simulink library "myLibrary"  (R2023a)
settings: Solver=VariableStepAuto  StartTime=0.0  StopTime=10.0  RelTol=1e-3
undefined symbols (not defined in the file): Cac_n1, ctrl1, Da, Discrete, dtha, ee_sli_rtmsupport, FA, gcbh, Ha, Ini, init_line, init_load, init_SG, init_TH, init_trafo, init_VSC, initMachineBlocks, Ka, Lf, Llkd_pu, Llkq1_pu, NET, P, plots_step, q0, Rac_n1, Radd, Rkd_pu, Rkq1_pu, Rload_add, sim_config, spsSteamTurbineModel, T_global, T_load, T_NET, T_SG, T_TH, T_trafo, T_VSC, Ts, tstep, V1
libraries: spsSeriesRLCBranchLib x57, spsParallelRLCBranchLib x39, eeGeneralControl x38, spsCurrentMeasurementLib x20, spsFirstOrderFilterLib x16, spsVoltageMeasurementLib x14, spsControlledVoltageSourceLib x12, $bdroot x9, dspsigops x6, spsThreePhaseVIMeasurementLib x5, spsPLL3phLib x4, spsThreePhaseBreakerLib x3
(part 3 of 7)

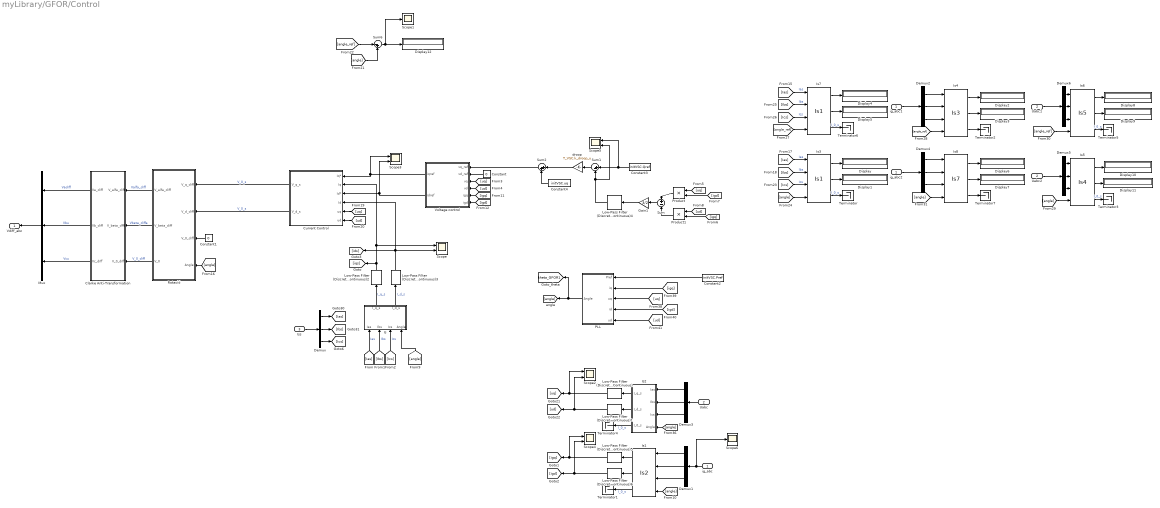
== system myLibrary/GFOR/Control ==
  ig_abc : Inport
  Uabc : Inport  Port=2
  Iss : Inport  Port=3
  Clarke Anti-Transformation : Subsystem
  Constant : Constant  Value=0
  Constant1 : Constant  Value=0
  Constant2 : Constant  Value=initVSC.Pref
  Constant3 : Constant  Value=initVSC.Qref
  Constant4 : Constant  Value=initVSC.uq
  Current Control : Subsystem
  Demux{,1..6} (7 alike) : Demux  Outputs=3
  Display{,1..12} (13 alike) : Display
  Gain1 : Gain  Gain=3/2
  Is : Subsystem
  Is1 : $bdroot/GFOR/Control/Is2  SystemSampleTime=-1  VariantActivationTime=update diagram  Latency=0  AutoFrameSizeCalculation=off
  Is2 : Subsystem
  Is3 : $bdroot/GFOL/Control/Is1  SystemSampleTime=-1  VariantActivationTime=update diagram  Latency=0  AutoFrameSizeCalculation=off
  Is4 : $bdroot/GFOL/Control/Is3  SystemSampleTime=-1  VariantActivationTime=update diagram  Latency=0  AutoFrameSizeCalculation=off
  Is5 : $bdroot/GFOL/Control/Is4  SystemSampleTime=-1  VariantActivationTime=update diagram  Latency=0  AutoFrameSizeCalculation=off
  Is6 : $bdroot/GFOL/Control/Is5  SystemSampleTime=-1  VariantActivationTime=update diagram  Latency=0  AutoFrameSizeCalculation=off
  Is7 : $bdroot/GFOL/Control/Is1  SystemSampleTime=-1  VariantActivationTime=update diagram  Latency=0  AutoFrameSizeCalculation=off
  Is8 : $bdroot/GFOL/Control/Is7  SystemSampleTime=-1  VariantActivationTime=update diagram  Latency=0  AutoFrameSizeCalculation=off
  Low-Pass Filter (Discrete or Continuous) : eeGeneralControl/Low-Pass Filter (Discrete or Continuous)  K=1  T=init_VSC.delay  B=inf  A=-inf  init_option=Specify as parameter  x0=initVSC.uq  Ts=0
  Low-Pass Filter (Discrete or Continuous)1 : eeGeneralControl/Low-Pass Filter (Discrete or Continuous)  K=1  T=init_VSC.delay  B=inf  A=-inf  init_option=Specify as parameter  x0=initVSC.ud  Ts=0
  Low-Pass Filter (Discrete or Continuous)2 : eeGeneralControl/Low-Pass Filter (Discrete or Continuous)  K=1  T=init_VSC.delay  B=inf  A=-inf  init_option=Specify as parameter  x0=initVSC.idiffq  Ts=0
  Low-Pass Filter (Discrete or Continuous)3 : eeGeneralControl/Low-Pass Filter (Discrete or Continuous)  K=1  T=init_VSC.delay  B=inf  A=-inf  init_option=Specify as parameter  x0=initVSC.idiffd  Ts=0
  Low-Pass Filter (Discrete or Continuous)4 : eeGeneralControl/Low-Pass Filter (Discrete or Continuous)  K=1  T=T_VSC.tau_droop_u  B=inf  A=-inf  init_option=Specify as parameter  x0=initVSC.Qref  Ts=0
  Low-Pass Filter (Discrete or Continuous)5 : eeGeneralControl/Low-Pass Filter (Discrete or Continuous)  K=1  T=init_VSC.delay  B=inf  A=-inf  init_option=Specify as parameter  x0=initVSC.igq  Ts=0
  Low-Pass Filter (Discrete or Continuous)6 : eeGeneralControl/Low-Pass Filter (Discrete or Continuous)  K=1  T=init_VSC.delay  B=inf  A=-inf  init_option=Specify as parameter  x0=initVSC.igd  Ts=0
  Mux : Mux  Inputs=3
  PLL : Subsystem
  Product : Product
  Product1 : Product
  Rotació : Subsystem
  Scope{,2..5} (5 alike) : Scope  NumInputPorts=2
  Scope1 : Scope
  Scope6 : Scope
  Sum : Sum  Inputs=+-
  Sum1 : Sum  Inputs=|+-
  Sum2 : Sum  Inputs=|++
  Sum6 : Sum  Inputs=|-+
  Terminator{,1..7} (8 alike) : Terminator
  Uabc1 : InportShadow  Port=2
  Uabc2 : InportShadow  Port=2
  Voltage control : Subsystem
  droop : Gain  Gain=T_VSC.k_droop_u
  ig_abc1 : InportShadow
  ig_abc2 : InportShadow
  Vdiff_abc : Outport
  tag scope: theta_GFOR1=global
  wires:
  Constant1/1 -> Rotació/3(V_0_diff)
  Low-Pass Filter (Discrete or Continuous)2/1 -> [iqs], Scope/1, Current Control/2(Iq)
  Low-Pass Filter (Discrete or Continuous)3/1 -> [ids], Current Control/4(Id), Scope/2
  Mux/1 -> Vdiff_abc/1
  Clarke Anti-Transformation/2(Vb_diff) -> Mux/2  "Vbu"
  Clarke Anti-Transformation/3(Vc_diff) -> Mux/3  "Vcu"
  Rotació/3(V_0) -> Clarke Anti-Transformation/3(V_0_diff)  "V_0_diff"
  Clarke Anti-Transformation/1(Va_diff) -> Mux/1  "Vadiff"
  Rotació/2(V_beta_diff) -> Clarke Anti-Transformation/2(V_beta_dfff)  "Vbeta_diffa"
  Rotació/1(V_alfa_diff) -> Clarke Anti-Transformation/1(V_alfa_diff)  "Valfa_diff"
  [angle_ref] -> Sum6/1
  Sum6/1 -> Display12/1, Scope1/1
  [angle] -> Sum6/2
  [ud] -> Current Control/6(ud)
  [uq] -> Current Control/5(uq)
  Current Control/2(V_d_s) -> Rotació/2(V_d_diff)  "V_0_s"
  Current Control/1(V_q_s) -> Rotació/1(V_q_diff)  "V_0_s"
  [angle] -> Rotació/4(Angle)
  [angle] -> Is/4(Angle)
  Iss/1 -> Demux/1
  Demux/3 -> [Ics]
  Demux/2 -> [Ibs]
  Demux/1 -> [Ias]
  [Ibs] -> Is/2(Ibs)  "Ibs"
  [Ics] -> Is/3(Ics)  "Ics"
  [Ias] -> Is/1(Ias)  "Ias"
  Is/1(I_q_s) -> Low-Pass Filter (Discrete or Continuous)2/1  "I_q_s"
  Is/2(I_d_s) -> Low-Pass Filter (Discrete or Continuous)3/1  "I_d_s"
  Constant/1 -> Voltage control/2(vd_ref)
  [igq] -> PLL/2(iq)
  Demux3/3 -> Is2/3(Ics)
  Demux3/2 -> Is2/2(Ibs)
  [angle] -> Is2/4(Angle)
  PLL/1(Angle) -> [theta_GFOR1], [angle]
  [uq] -> Voltage control/3(vq)
  [igd] -> PLL/4(id)
  Demux3/1 -> Is2/1(Ias)
  Low-Pass Filter (Discrete or Continuous)/1 -> Scope2/1, [uq]
  [uq] -> PLL/3(uq)
  Sum2/1 -> Voltage control/1(vq_ref)
  Constant2/1 -> PLL/1(Pref)
  [ud] -> Voltage control/4(vd)
  Low-Pass Filter (Discrete or Continuous)1/1 -> [ud], Scope2/2
  Is2/3(I_0_s) -> Terminator4/1  "I_0_s"
  Is2/2(I_d_s) -> Low-Pass Filter (Discrete or Continuous)1/1
  Uabc/1 -> Demux3/1
  Is2/1(I_q_s) -> Low-Pass Filter (Discrete or Continuous)/1
  [ud] -> PLL/5(ud)
  Voltage control/1(iqref) -> Current Control/1(Iq*), Scope3/1
  Voltage control/2(idref) -> Scope3/2, Current Control/3(Id*)
  [igd] -> Product/2
  Constant3/1 -> Sum1/1, Scope5/1
  Gain1/1 -> Low-Pass Filter (Discrete or Continuous)4/1
  Product1/1 -> Sum/2
  Product/1 -> Sum/1
  Sum/1 -> Gain1/1
  [igq] -> Product1/2
  Constant4/1 -> Sum2/2
  Sum1/1 -> droop/1
  [uq] -> Product/1
  [ud] -> Product1/1
  droop/1 -> Sum2/1
  Low-Pass Filter (Discrete or Continuous)4/1 -> Sum1/2, Scope5/2
  Low-Pass Filter (Discrete or Continuous)5/1 -> Scope4/1, [igq]
  Demux1/1 -> Is1/1
  Demux1/3 -> Is1/3
  ig_abc/1 -> Demux1/1, Scope6/1
  Is1/3 -> Terminator1/1  "I_0_s"
  Demux1/2 -> Is1/2
  Is1/2 -> Low-Pass Filter (Discrete or Continuous)6/1
  [angle] -> Is1/4
  Low-Pass Filter (Discrete or Continuous)6/1 -> [igd], Scope4/2
  Is1/1 -> Low-Pass Filter (Discrete or Continuous)5/1
  [igq] -> Voltage control/5(igq)
  [igd] -> Voltage control/6(igd)
  [angle] -> Is8/4
  Is4/2 -> Display3/1
  Is8/1 -> Display6/1
  Demux5/1 -> Is5/1
  [Ics] -> Is3/3  "Ics"
  Is8/3 -> Terminator7/1
  Uabc2/1 -> Demux5/1
  Demux2/3 -> Is4/3
  Demux2/1 -> Is4/1
  Is5/2 -> Display11/1
  Demux6/1 -> Is6/1
  Is5/3 -> Terminator3/1  "I_0_s"
  Demux6/3 -> Is6/3
  Is4/1 -> Display2/1
  ig_abc1/1 -> Demux2/1
  Demux4/3 -> Is8/3
  [Ias] -> Is7/1  "Ias"
  [Ibs] -> Is7/2  "Ibs"
  Demux5/2 -> Is5/2
  ig_abc2/1 -> Demux4/1
  Demux5/3 -> Is5/3
  Is7/3 -> Terminator6/1  "I_0_s"
  [angle_ref] -> Is4/4
  Is3/1 -> Display/1
  [Ics] -> Is7/3  "Ics"
  [angle_ref] -> Is7/4
  Is8/2 -> Display7/1
  Is7/2 -> Display5/1
  Is6/1 -> Display8/1
  Demux2/2 -> Is4/2
  [angle_ref] -> Is6/4
  [angle] -> Is3/4
  Is6/3 -> Terminator5/1  "I_0_s"
  Is4/3 -> Terminator2/1
  Is5/1 -> Display10/1
  Is7/1 -> Display4/1
  Demux4/1 -> Is8/1
  [Ias] -> Is3/1  "Ias"
  [Ibs] -> Is3/2  "Ibs"
  Is3/2 -> Display1/1
  Uabc1/1 -> Demux6/1
  Is6/2 -> Display9/1
  [angle] -> Is5/4
  Demux6/2 -> Is6/2
  Demux4/2 -> Is8/2
  Is3/3 -> Terminator/1  "I_0_s"

== system myLibrary/GFOR/Electrical ==
  note: DIFF CIRCUIT:
  Vdiff : Inport
  Controlled Voltage Source1 : spsControlledVoltageSourceLib/Controlled Voltage Source  Initialize=on  Source_Type=AC  Amplitude=initVSC.Udiff_mag  Phase=initVSC.angle_vdiff*180/pi  Frequency=T_VSC.fb  Measurements=None
  Controlled Voltage Source2 : spsControlledVoltageSourceLib/Controlled Voltage Source  Initialize=on  Source_Type=AC  Amplitude=initVSC.Udiff_mag  Phase=(initVSC.angle_vdiff -2*pi/3)*180/pi  Frequency=T_VSC.fb  Measurements=None
  Controlled Voltage Source3 : spsControlledVoltageSourceLib/Controlled Voltage Source  Initialize=on  Source_Type=AC  Amplitude=initVSC.Udiff_mag  Phase=(initVSC.angle_vdiff +2*pi/3)*180/pi  Frequency=T_VSC.fb  Measurements=None
  Demux : Demux  Outputs=3
  Mesura Ias10 : spsCurrentMeasurementLib/Current Measurement  PhasorSimulation=off  OutputType=Complex  PSBequivalent=0
  Mesura Ias7 : spsCurrentMeasurementLib/Current Measurement  PhasorSimulation=off  OutputType=Complex  PSBequivalent=0
  Mesura Ias9 : spsCurrentMeasurementLib/Current Measurement  PhasorSimulation=off  OutputType=Complex  PSBequivalent=0
  Mux : Mux  Inputs=3
  Scope : Scope
  Scope10 : Scope  NumInputPorts=3
  Zsa : spsSeriesRLCBranchLib/Series RLC Branch  LConnTagsString=__new0  RConnTagsString=__new0  BranchType=RL  Resistance=initVSC.Rc  Inductance=initVSC.Lc  SetiL0=off  InitialCurrent=initVSC.Isa  Capacitance=1e-6  Setx0=off  InitialVoltage=0  Measurements=None
  Zsa1 : spsSeriesRLCBranchLib/Series RLC Branch  LConnTagsString=__new0  RConnTagsString=__new0  BranchType=RL  Resistance=initVSC.Rc  Inductance=initVSC.Lc  SetiL0=on  InitialCurrent=initVSC.Isb  Capacitance=1e-6  Setx0=off  InitialVoltage=0  Measurements=None
  Zsa2 : spsSeriesRLCBranchLib/Series RLC Branch  LConnTagsString=__new0  RConnTagsString=__new0  BranchType=RL  Resistance=initVSC.Rc  Inductance=initVSC.Lc  SetiL0=on  InitialCurrent=initVSC.Isc  Capacitance=1e-6  Setx0=off  InitialVoltage=0  Measurements=None
  VA : PMIOPort  Side=Left
  VB : PMIOPort  Port=2  Side=Left
  VC : PMIOPort  Port=3  Side=Left
  Is : Outport
  wires:
  Mesura Ias10/1 -> [Ics]
  Mesura Ias7/1 -> [Ias]
  Mesura Ias9/1 -> [Ibs]
  Vdiff/1 -> Demux/1
  Demux/1 -> [Vdiffa]
  Demux/3 -> [Vdiffc]
  Demux/2 -> [Vdiffb]
  Mux/1 -> Scope/1, Is/1
  [Ics] -> Mux/3  "Ics"
  [Ibs] -> Mux/2  "Ibs"
  [Ias] -> Mux/1  "Ias"
  [Vdiffa] -> Controlled Voltage Source1/1, Scope10/1
  [Vdiffb] -> Scope10/2, Controlled Voltage Source2/1
  [Vdiffc] -> Controlled Voltage Source3/1, Scope10/3
  connections:
  Zsa1/LConn1 -- Controlled Voltage Source2/RConn1
  Mesura Ias7/RConn1 -- VA/RConn1
  Mesura Ias9/RConn1 -- VB/RConn1
  Mesura Ias10/RConn1 -- VC/RConn1
  Zsa/RConn1 -- Mesura Ias7/LConn1
  Zsa1/RConn1 -- Mesura Ias9/LConn1
  Zsa2/RConn1 -- Mesura Ias10/LConn1
  Controlled Voltage Source1/RConn1 -- Zsa/LConn1
  Zsa2/LConn1 -- Controlled Voltage Source3/RConn1
  Controlled Voltage Source3/LConn1 -- Controlled Voltage Source1/LConn1 -- Controlled Voltage Source2/LConn1

== system myLibrary/SG/Exciter ==
  V_REF : Inport
  Vq : Inport  Port=2
  Vd : Inport  Port=3
  Vsi1 : Inport  Port=4
  Vsi2 : Inport  Port=5
  Ifd_pu : Inport  Port=6
  Efd0_pu : Inport  Port=7
  Constant : Constant  Value=hasPSS
  Constant1 : Constant  Value=selectExciter
  Constant4 : Constant
  Constant5 : Constant  Value=initSG.Pm
  Exciter AC4A : Subsystem
  Exciter ST1 : Subsystem  Commented=on
  Exciter ST4B : Subsystem  Commented=on  AncestorBlock=eeSmST4C/SM ST4C  LoadFcn=ee_sli_rtmsupport( 'loadfcn', gcbh );  mask(SM ST4C){E_FD0=1, V_T0=1, I_T0=1, Ts=-1, T_R=T_SG.exc.TR, K_PR=T_SG.exc.KPR, K_IR=T_SG.exc.KIR, T_A=T_SG.exc.TA, K_PM=T_SG.exc.KPM, K_IM=T_SG.exc.KIM, K_G=T_SG.exc.KG, T_G=0, K_C=T_SG.exc.KC, K_P=T_SG.exc.KP, K_I=T_SG.exc.KI, X_L=T_SG.exc.XL, theta_P=0}
      mask prompts: E_FD0 "physmod:ee:library:comments:control:eeSmST4C:InitialFieldVoltageEfd0pu_MP"; V_T0 "physmod:ee:library:comments:control:eeSmST4C:InitialTerminalVoltageVt0pu_MP"; I_T0 "physmod:ee:library:comments:control:eeSmST4C:InitialTerminalCurrentIt0pu_MP"; Ts "physmod:ee:library:comments:control:eeSmST4C:SampleTime1ForInherited_MP"; T_R "physmod:ee:library:comments:control:eeSmST4C:RegulatorInputFilterTimeConstantT_Rs_MP"; K_PR "physmod:ee:library:comments:control:eeSmST4C:VoltageRegulatorProportionalGainK_PRpu_MP"; K_IR "physmod:ee:library:comments:control:eeSmST4C:VoltageRegulatorIntegralGainK_IRpus_MP"; T_A "physmod:ee:library:comments:control:eeSmST4C:ThyristorBridgeFiringControlEquivalentTimeConstantT_As_MP"; K_PM "physmod:ee:library:comments:control:eeSmST4C:ForwardProportionalGainOfInnerLoopFieldRegulatorK_PMpu_MP"; K_IM "physmod:ee:library:comments:control:eeSmST4C:ForwardIntegralGainOfInnerLoopFieldRegulatorK_IMpus_MP"; K_G "physmod:ee:library:comments:control:eeSmST4C:FeedbackGainOfFieldCurrentRegulatorK_Gpu_MP"; T_G "physmod:ee:library:comments:control:eeSmST4C:FeedbackTimeConstantOfFieldCurrentRegulatorT_Gs_MP"; K_C "physmod:ee:library:comments:control:eeSmST4C:RectifierLoadingFactorProportionalToCommutatingReactanceK_Cp_MP"; K_P "physmod:ee:library:comments:control:eeSmST4C:PotentialCircuitvoltageGainCoefficientK_Ppu_MP"; K_I "physmod:ee:library:comments:control:eeSmST4C:CompoundCircuitcurrentGainCoefficientK_Ipu_MP"; X_L "physmod:ee:library:comments:control:eeSmST4C:ReactanceAssociatedWithPotentialSourceX_Lpu_MP"; theta_P "physmod:ee:library:comments:control:eeSmST4C:PotentialCircuitPhaseAngledegrees_MP"
      mask help: physmod:ee:library:comments:control:eeSmST4C:SMST4C_MD
      mask init:
      | %[timeDomain,isVsSummationPoint1,isVsSummationPoint2,...
      | %    isOelSummationPoint,isOelTakeOver1,isOelTakeOver2,...
      | %    isUelSummationPoint,isUelTakeOver1,isUelTakeOver2,...
      | %    isSclSummationPoint,isSclTakeOver1,isSclTakeOver2,isSw1LocationA]...
      | %    = ee.mask.initializeST4C(Ts,oelInputLocation,...
      | %    uelInputLocation,sclInputLocation,vsInputLocation,SW1);
      | 
      | %This will move to Initialization Function
      | %[V_G0,initialOffset] = ee.control.sm.initializeST4C(E_FD0,V_T0,I_T0,K_G,theta_P,K_P,X_L,K_I,K_C,V_Bmax,SW1);
      settings: LibrarySourceBlock=eeSmST4C/SM ST4C  CopyFcn=ee_sli_rtmsupport( 'copyfcn', gcbh );  DeleteFcn=ee_sli_rtmsupport( 'deletefcn', gcbh );  ModelCloseFcn=ee_sli_rtmsupport( 'modelclosefcn', gcbh );  PostSaveFcn=ee_sli_rtmsupport( 'postsavefcn', gcbh );  PreCopyFcn=ee_sli_rtmsupport( 'precopyfcn', gcbh );  OpenFcn=ee_sli_rtmsupport( 'openfcn', gcbh );  CloseFcn=ee_sli_rtmsupport( 'closefcn', gcbh );  PreDeleteFcn=ee_sli_rtmsupport( 'predeletefcn', gcbh );
      mask Help: web(nesl_help(gcbh))
      mask TypeOptions Ts:
      | Voltage Transducer/Ts | PI_R/Integrator
      | (Discrete or Continuous)/Ts | PI_M/Integrator
      | (Discrete or Continuous)/Ts | VRminmax/Ts | K_G//(1+sT_G)/Ts
      mask DialogControl TabGeneral Prompt: physmod:ee:library:comments:control:eeSmST4C:tab_General
      mask DialogControl E_FD0 Prompt: Initial field voltage, Efd0 (pu)
      mask DialogControl V_T0 Prompt: Initial terminal voltage, Vt0 (pu)
      mask DialogControl I_T0 Prompt: Initial terminal current, It0 (pu)
      mask DialogControl Ts Prompt: Sample time (-1 for inherited)
      mask DialogControl TabPrecontrol Prompt: physmod:ee:library:comments:control:eeSmST4C:tab_PreControl
      mask DialogControl T_R Prompt: Regulator input filter time constant, T_R (s)
      mask DialogControl TabControl Prompt: physmod:ee:library:comments:control:eeSmST4C:tab_Control
      mask DialogControl K_PR Prompt: Voltage regulator proportional gain, K_PR (pu)
      mask DialogControl K_IR Prompt: Voltage regulator integral gain, K_IR (pu/s)
      mask DialogControl T_A Prompt: Thyristor bridge firing control equivalent time constant, T_A (s)
      mask DialogControl K_PM Prompt: Forward proportional gain of inner loop field regulator, K_PM (pu)
      mask DialogControl K_IM Prompt: Forward integral gain of inner loop field regulator, K_IM (pu/s)
      mask DialogControl K_G Prompt: Feedback gain of field current regulator, K_G (pu)
      mask DialogControl T_G Prompt: Feedback time constant of field current regulator, T_G (s)
      mask DialogControl TabExciter Prompt: physmod:ee:library:comments:control:eeSmST4C:tab_Exciter
      mask DialogControl K_C Prompt: Rectifier loading factor proportional to commutating reactance, K_C (pu)
      mask DialogControl K_P Prompt: Potential circuit (voltage) gain coefficient, K_P (pu)
      mask DialogControl K_I Prompt: Compound circuit (current) gain coefficient, K_I (pu)
      mask DialogControl X_L Prompt: Reactance associated with potential source, X_L (pu)
      mask DialogControl theta_P Prompt: Potential circuit phase angle (degrees)
      mask Display: %ee.mask.drawSTxC(gcb);
  Gain : Gain  Gain=T_SG.Lmd_pu
  Multiport Switch : MultiPortSwitch  Inputs=4  SaturateOnIntegerOverflow=off  InputSameDT=off
  PSS 2A : Subsystem  Commented=on  mask{ks1=T_SG.PSS.Ks1, ks2=T_SG.PSS.Ks2, ks3=T_SG.PSS.Ks3, T6=T_SG.PSS.T6, T7=T_SG.PSS.T7, Tw1=T_SG.PSS.Tw1, Tw2=T_SG.PSS.Tw2, Tw3=T_SG.PSS.Tw3, Tw4=T_SG.PSS.Tw4, T8=T_SG.PSS.T8, T9=T_SG.PSS.T9, M=T_SG.PSS.M, N=T_SG.PSS.N, T1=T_SG.PSS.T1, T2=T_SG.PSS.T2, T3=T_SG.PSS.T3, T4=T_SG.PSS.T4, hasPSS=hasPSS}
      mask prompts: ks1 "PSS gain, K_S1 (pu)"; ks2 "PSS gain, K_S2 (pu)"; ks3 "PSS gain, K_S3 (pu)"; T6 "PSS transducer time constant, T_6 (s)"; T7 "PSS transducer time constant, T_7 (s)"; Tw1 "PSS washout time constant, T_w1 (s)"; Tw2 "PSS washout time constant, T_w2 (s)"; Tw3 "PSS washout time constant, T_w3 (s)"; Tw4 "PSS washout time constant, T_w4 (s)"; T8 "PSS transducer time constant, T_8 (s)"; T9 "PSS washout time constant, T_9 (s)"; M "Denominator exponent for ramp-track filter, M"; N "Overall exponent for ramp-track filter, N"; T1 "PSS numerator (lead) compensating time constant (first block), T_1 (s)"; T2 "PSS denominator (lag) compensating time constant (first block), T_2 (s)"; T3 "PSS numerator (lead) compensating time constant (second block), T_3 (s)"; T4 "PSS denominator (lag) compensating time constant (second block), T_4 (s)"
      mask init:
      | if hasPSS == 1
      |     pss.Ks1 = 0;
      |     % TO BE CONTINUED
      | end
  Sum : Sum  Inputs=|++
  Sum1 : Sum  Inputs=|++
  Sum2 : Sum  Inputs=|++
  Sum3 : Sum  Inputs=|+-
  Sum6 : Sum  Inputs=|+-
  Switch : Switch  Threshold=1  SaturateOnIntegerOverflow=off  InputSameDT=off
  Terminal voltage magnitude : Subsystem
  Vst : Constant  Value=0
  Out1 : Outport
  wires:
  Constant5/1 -> Sum3/2
  Constant4/1 -> Sum6/2
  Sum3/1 -> PSS 2A/2(Vsi2)  "delta_Te_pu"
  Sum6/1 -> PSS 2A/1(Vsi1)  "delta_w_pu"
  Terminal voltage magnitude/1(Vt) -> Exciter ST1/2(Vt), Exciter ST4B/3(V_T), Exciter AC4A/2(Vt)
  Sum2/1 -> Multiport Switch/4
  Sum1/1 -> Multiport Switch/3
  Sum/1 -> Multiport Switch/2
  Multiport Switch/1 -> Out1/1
  Vd/1 -> Terminal voltage magnitude/2(Vd)
  Ifd_pu/1 -> Gain/1
  Exciter ST1/1(Vfn_pu) -> Sum2/1
  Exciter ST4B/1(Efd_pu) -> Sum1/1
  Constant/1 -> Switch/2
  Vsi2/1 -> Sum3/1
  Exciter AC4A/1(Vfn_pu) -> Sum/1
  Efd0_pu/1 -> Multiport Switch/5, Sum/2, Sum1/2, Sum2/2
  Vq/1 -> Terminal voltage magnitude/1(Vq)
  Vst/1 -> Switch/3  "Vst"
  Switch/1 -> Exciter ST1/3(Vs), Exciter AC4A/3(Vs), Exciter ST4B/2(V_S)
  Vsi1/1 -> Sum6/1
  PSS 2A/1(Vst) -> Switch/1  "Vst"
  V_REF/1 -> Exciter AC4A/1(vref), Exciter ST1/1(vref), Exciter ST4B/1(V_REF)
  Constant1/1 -> Multiport Switch/1
  Gain/1 -> Exciter ST4B/4(Ifd_pu)

== system myLibrary/SG/Governor-Turbine ==
  Pref : Inport
  wm : Inport  Port=2
  d_theta : Inport  Port=3
  Constant : Constant  Value=selectGovturb
  IEEEG1 : Subsystem  AncestorBlock=eeGovernorG1/Governor Type 1  LoadFcn=ee_sli_rtmsupport( 'loadfcn', gcbh );  mask(Governor Type 1){pu_speed_reference=1, pu_torque0=initSG.Pm, Ts=-1, K=1/T_SG.mech.R, T_1=initMachineBlocks{SGnum,14}(1), T_2=initMachineBlocks{SGnum,14}(2), T_3=initMachineBlocks{SGnum,14}(3), U_o=inf, U_c=-inf, P_max=1, P_min=0, K_1=initMachineBlocks{SGnum,15}(1), K_3=initMachineBlocks{SGnum,15}(2), K_5=initMachineBlocks{SGnum,15}(3), K_7=initMachineBlocks{SGnum,15}(4), K_2=initMachineBlocks{SGnum,15}(5), K_4=initMachineBlocks{SGnum,15}(6), K_6=initMachineBlocks{SGnum,15}(7), K_8=initMachineBlocks{SGnum,15}(8), T_4=initMachineBlocks{SGnum,15}(9), T_5=initMachineBlocks{SGnum,15}(10), T_6=initMachineBlocks{SGnum,15}(11), T_7=initMachineBlocks{SGnum,15}(12), db1=1}
      mask prompts: pu_speed_reference "physmod:ee:library:comments:control:eeGovernorG1:SpeedReferencepu_MP"; pu_torque0 "physmod:ee:library:comments:control:eeGovernorG1:InitialTorquepu_MP"; Ts "physmod:ee:library:comments:control:eeGovernorG1:SampleTime1ForInherited_MP"; K "physmod:ee:library:comments:control:eeGovernorG1:GovernorGain1droopKpu_MP"; T_1 "physmod:ee:library:comments:control:eeGovernorG1:LagTimeConstantT_1s_MP"; T_2 "physmod:ee:library:comments:control:eeGovernorG1:LeadTimeConstantT_2s_MP"; T_3 "physmod:ee:library:comments:control:eeGovernorG1:ValvePositionTimeConstantT_3s_MP"; U_o "physmod:ee:library:comments:control:eeGovernorG1:MaximumValveOpeningRateU_opus_MP"; U_c "physmod:ee:library:comments:control:eeGovernorG1:MaximumValveClosingRateU_cpus_MP"; P_max "physmod:ee:library:comments:control:eeGovernorG1:MaximumValveOpeningOnMWCapabilityP_maxpu_MP"; P_min "physmod:ee:library:comments:control:eeGovernorG1:MinimumValveOpeningOnMWCapabilityP_minpu_MP"; K_1 "physmod:ee:library:comments:control:eeGovernorG1:HPFractionK_1_MP"; K_3 "physmod:ee:library:comments:control:eeGovernorG1:HPFractionK_3_MP"; K_5 "physmod:ee:library:comments:control:eeGovernorG1:HPFractionK_5_MP"; K_7 "physmod:ee:library:comments:control:eeGovernorG1:HPFractionK_7_MP"; K_2 "physmod:ee:library:comments:control:eeGovernorG1:LPFractionK2_MP"; K_4 "physmod:ee:library:comments:control:eeGovernorG1:LPFractionK_4_MP"; K_6 "physmod:ee:library:comments:control:eeGovernorG1:LPFractionK_6_MP"; K_8 "physmod:ee:library:comments:control:eeGovernorG1:LPFractionK_8_MP"; T_4 "physmod:ee:library:comments:control:eeGovernorG1:TimeConstantForSteamInletT_4s_MP"; T_5 "physmod:ee:library:comments:control:eeGovernorG1:TimeConstantForSecondBoilerPassT_5s_MP"; T_6 "physmod:ee:library:comments:control:eeGovernorG1:TimeConstantForThirdBoilerPassT_6s_MP"; T_7 "physmod:ee:library:comments:control:eeGovernorG1:TimeConstantForFourthBoilerPassT_7s_MP"; db1 "physmod:ee:library:comments:control:eeGovernorG1:Deadband_MP"
      mask help: physmod:ee:library:comments:control:eeGovernorG1:GovernorType1_MD
      mask init:
      | timeDomain = ee.mask.getTimeDomain(Ts);
      settings: LibrarySourceBlock=eeGovernorG1/Governor Type 1  CopyFcn=ee_sli_rtmsupport( 'copyfcn', gcbh );  DeleteFcn=ee_sli_rtmsupport( 'deletefcn', gcbh );  ModelCloseFcn=ee_sli_rtmsupport( 'modelclosefcn', gcbh );  PostSaveFcn=ee_sli_rtmsupport( 'postsavefcn', gcbh );  PreCopyFcn=ee_sli_rtmsupport( 'precopyfcn', gcbh );  OpenFcn=ee_sli_rtmsupport( 'openfcn', gcbh );  CloseFcn=ee_sli_rtmsupport( 'closefcn', gcbh );  PreDeleteFcn=ee_sli_rtmsupport( 'predeletefcn', gcbh );
      mask Help: web(nesl_help(gcbh))
      mask TypeOptions Ts:
      | Lead-Lag/Ts | Low-Pass Filter/Ts | Low-Pass Filter1/Ts | Low-Pass Filter2/Ts | Low-Pass Filter3/Ts | Integrator
      | (Discrete or Continuous)/Ts
      mask DialogControl TabGeneral Prompt: physmod:ee:library:comments:control:eeGovernorG1:tab_General
      mask DialogControl pu_speed_reference Prompt: Speed reference (pu)
      mask DialogControl pu_torque0 Prompt: Initial torque (pu)
      mask DialogControl Ts Prompt: Sample time (-1 for inherited)
      mask DialogControl TabGovernor Prompt: physmod:ee:library:comments:control:eeGovernorG1:tab_Governor
      mask DialogControl K Prompt: Governor gain (1/droop), K (pu)
      mask DialogControl T_1 Prompt: Lag time constant, T_1 (s)
      mask DialogControl T_2 Prompt: Lead time constant, T_2 (s)
      mask DialogControl T_3 Prompt: Valve position time constant, T_3 (s)
      mask DialogControl U_o Prompt: Maximum valve opening rate, U_o (pu/s)
      mask DialogControl U_c Prompt: Maximum valve closing rate, U_c (pu/s)
      mask DialogControl P_max Prompt: Maximum valve opening, on MW capability, P_max (pu)
      mask DialogControl P_min Prompt: Minimum valve opening, on MW capability, P_min (pu)
      mask DialogControl K_1 Prompt: HP fraction, K_1
      mask DialogControl K_3 Prompt: HP fraction, K_3
      mask DialogControl K_5 Prompt: HP fraction, K_5
      mask DialogControl K_7 Prompt: HP fraction, K_7
      mask DialogControl K_2 Prompt: LP fraction, K2
      mask DialogControl K_4 Prompt: LP fraction, K_4
      mask DialogControl K_6 Prompt: LP fraction, K_6
      mask DialogControl K_8 Prompt: LP fraction, K_8
      mask DialogControl T_4 Prompt: Time constant for steam inlet, T_4 (s)
      mask DialogControl T_5 Prompt: Time constant for second boiler pass, T_5 (s)
      mask DialogControl T_6 Prompt: Time constant for third boiler pass, T_6 (s)
      mask DialogControl T_7 Prompt: Time constant for fourth boiler pass, T_7 (s)
      mask DialogControl db1 Prompt: Deadband
  Multiport Switch1 : MultiPortSwitch  SaturateOnIntegerOverflow=off  InputSameDT=off
  Steam Turbine and Governor : Subsystem  Commented=on  DialogController=POWERSYS.PowerSysDialog  mask(Steam Turbine and Governor){gentype=Tandem-compound (multi-mass), reg1=[ 1  T_SG.mech.R   0 ], reg2=[ 0  1], reg3=[ -inf  inf  0  inf], N=T_SG.fb*60, turb1=initMachineBlocks{SGnum,8}, turb2=initMachineBlocks{SGnum,9}, HA=initMachineBlocks{SGnum,10}, KA=initMachineBlocks{SGnum,11}, DA=initMachineBlocks{SGnum,12}, ini1=1.003, ini2=initMachineBlocks{SGnum,7}}
      mask prompts: gentype "Generator type"; reg1 "Regulator gain, perm. droop, dead zone [ Kp  Rp(pu)  Dz(pu) ]:"; reg2 "Speed relay and servo-motor time constants [ Tsr  Tsm ] (s):"; reg3 "Gate opening limits [ vgmin,vgmax (pu/s)  gmin,gmax (pu)]:"; N "Nominal speed of synchronous machine (rpm)"; turb1 "Steam turbine time constants [ T2  T3  T4  T5 ] (s):"; turb2 "Turbine torque fractions [ F2  F3  F4  F5 ]:"; HA "Coeff. of inertia [ H2  H3  H4  H5 ] (s):"; KA "Stiffness coeff. [ K12  K23  K34  K45 ] (pu/rad):"; DA "Damping factors [ D2  D3  D4  D5 ] (pu T/pu dw):"; ini1 "Initial power Pm0 (pu):"; ini2 "Initial power and generator rotor angle [ Pm0 (pu)  th0(deg) ]:"
      mask help:
      | Implements a complete tandem-compound steam prime mover system, including
      | speed regulator, steam turbine and a shaft with up to 4 masses. The genererator's
      | mass is labelled mass #1 and is not included here. The shaft mass closest to the
      | generator is #2, the farthest is #5. If a mass is not to be included, set it's inertia H to
      | zero. The damping factor and rigidity coefficients corresponding to omitted masses
      | are not considered and can be left as is. When masses are omitted, the remaining
      | system is "compressed" towards the generator i.e. if only 2 masses are used, it will
      | be masses #2 and #3. The input data for the masses considered is shifted accordingly.
      mask init:
      | block = gcb;
      | [Ts, WantBlockChoice, q0,FA,Ha,Ka,Da,dtha,t,errorFlag,ctrl1,sel,massNumber] = powericon('SteamTurbineInit',gcb,gentype,reg1,reg2,reg3,turb1,turb2,HA,KA,DA,ini1,ini2);
      | %powericon('SetInternalModels','set',block,WantBlockChoice);
      settings: OpenFcn=sps_rtmsupport('OpenFcn',gcbh)
      mask Help: helpview(psbhelp);
      mask TypeOptions gentype: Tandem-compound (single mass) | Tandem-compound (multi-mass)
      mask Callback gentype: powericon('psbcallbacks',gcbh,'SteamTurbine');
      mask Display: %plot([0 0],[t t])
  Terminator1 : Terminator
  Terminator2 : Terminator
  Terminator3 : Terminator  Commented=on
  Terminator4 : Terminator  Commented=on
  Terminator5 : Terminator  Commented=on
  w_ref : Constant
  Pm : Outport
  wires:
  Steam Turbine and Governor/4(Pm) -> Multiport Switch1/3  "Pm"
  Steam Turbine and Governor/1(dw_5-2) -> Terminator5/1
  Steam Turbine and Governor/3(gate) -> Terminator3/1
  Steam Turbine and Governor/2(Tr5-2) -> Terminator4/1
  w_ref/1 -> Steam Turbine and Governor/1(wref)
  d_theta/1 -> Steam Turbine and Governor/4(d_theta)
  wm/1 -> Steam Turbine and Governor/3(wm), IEEEG1/1(speed_pu)
  IEEEG1/3(Pm) -> Multiport Switch1/2
  Constant/1 -> Multiport Switch1/1
  Multiport Switch1/1 -> Pm/1
  IEEEG1/2(Pm(LP)) -> Terminator2/1
  IEEEG1/1(Pm(HP)) -> Terminator1/1
  Pref/1 -> IEEEG1/2(Pref), Steam Turbine and Governor/2(Pref), Multiport Switch1/4

== system myLibrary/SG/Vector magnitude  ==
  Vq : Inport
  Vd : Inport  Port=2
  Add10 : Sum
  Product : Product
  Product1 : Product
  Square Root : Sqrt
  V : Outport
  wires:
  Square Root/1 -> V/1  "V"
  Vq/1 -> Product/2, Product/1
  Add10/1 -> Square Root/1
  Product1/1 -> Add10/2
  Vd/1 -> Product1/1, Product1/2
  Product/1 -> Add10/1

== system myLibrary/SG_step/Exciter ==
  V_REF : Inport
  Vq : Inport  Port=2
  Vd : Inport  Port=3
  Vsi1 : Inport  Port=4
  Vsi2 : Inport  Port=5
  Ifd_pu : Inport  Port=6
  Efd0_pu : Inport  Port=7
  Constant : Constant  Value=hasPSS
  Constant1 : Constant  Value=selectExciter
  Constant4 : Constant
  Constant5 : Constant  Value=initSG.Pm
  Exciter AC4A : Subsystem
  Exciter ST1 : Subsystem  Commented=on
  Exciter ST4B : Subsystem  Commented=on  AncestorBlock=eeSmST4C/SM ST4C  LoadFcn=ee_sli_rtmsupport( 'loadfcn', gcbh );  mask(SM ST4C){E_FD0=1, V_T0=1, I_T0=1, Ts=-1, T_R=T_SG.exc.TR, K_PR=T_SG.exc.KPR, K_IR=T_SG.exc.KIR, T_A=T_SG.exc.TA, K_PM=T_SG.exc.KPM, K_IM=T_SG.exc.KIM, K_G=T_SG.exc.KG, T_G=0, K_C=T_SG.exc.KC, K_P=T_SG.exc.KP, K_I=T_SG.exc.KI, X_L=T_SG.exc.XL, theta_P=0}
      mask prompts: E_FD0 "physmod:ee:library:comments:control:eeSmST4C:InitialFieldVoltageEfd0pu_MP"; V_T0 "physmod:ee:library:comments:control:eeSmST4C:InitialTerminalVoltageVt0pu_MP"; I_T0 "physmod:ee:library:comments:control:eeSmST4C:InitialTerminalCurrentIt0pu_MP"; Ts "physmod:ee:library:comments:control:eeSmST4C:SampleTime1ForInherited_MP"; T_R "physmod:ee:library:comments:control:eeSmST4C:RegulatorInputFilterTimeConstantT_Rs_MP"; K_PR "physmod:ee:library:comments:control:eeSmST4C:VoltageRegulatorProportionalGainK_PRpu_MP"; K_IR "physmod:ee:library:comments:control:eeSmST4C:VoltageRegulatorIntegralGainK_IRpus_MP"; T_A "physmod:ee:library:comments:control:eeSmST4C:ThyristorBridgeFiringControlEquivalentTimeConstantT_As_MP"; K_PM "physmod:ee:library:comments:control:eeSmST4C:ForwardProportionalGainOfInnerLoopFieldRegulatorK_PMpu_MP"; K_IM "physmod:ee:library:comments:control:eeSmST4C:ForwardIntegralGainOfInnerLoopFieldRegulatorK_IMpus_MP"; K_G "physmod:ee:library:comments:control:eeSmST4C:FeedbackGainOfFieldCurrentRegulatorK_Gpu_MP"; T_G "physmod:ee:library:comments:control:eeSmST4C:FeedbackTimeConstantOfFieldCurrentRegulatorT_Gs_MP"; K_C "physmod:ee:library:comments:control:eeSmST4C:RectifierLoadingFactorProportionalToCommutatingReactanceK_Cp_MP"; K_P "physmod:ee:library:comments:control:eeSmST4C:PotentialCircuitvoltageGainCoefficientK_Ppu_MP"; K_I "physmod:ee:library:comments:control:eeSmST4C:CompoundCircuitcurrentGainCoefficientK_Ipu_MP"; X_L "physmod:ee:library:comments:control:eeSmST4C:ReactanceAssociatedWithPotentialSourceX_Lpu_MP"; theta_P "physmod:ee:library:comments:control:eeSmST4C:PotentialCircuitPhaseAngledegrees_MP"
      mask help: physmod:ee:library:comments:control:eeSmST4C:SMST4C_MD
      mask init: same as myLibrary/SG/Exciter/Exciter ST4B
      settings: LibrarySourceBlock=eeSmST4C/SM ST4C  CopyFcn=ee_sli_rtmsupport( 'copyfcn', gcbh );  DeleteFcn=ee_sli_rtmsupport( 'deletefcn', gcbh );  ModelCloseFcn=ee_sli_rtmsupport( 'modelclosefcn', gcbh );  PostSaveFcn=ee_sli_rtmsupport( 'postsavefcn', gcbh );  PreCopyFcn=ee_sli_rtmsupport( 'precopyfcn', gcbh );  OpenFcn=ee_sli_rtmsupport( 'openfcn', gcbh );  CloseFcn=ee_sli_rtmsupport( 'closefcn', gcbh );  PreDeleteFcn=ee_sli_rtmsupport( 'predeletefcn', gcbh );
      mask Help: web(nesl_help(gcbh))
      mask TypeOptions Ts:
      | Voltage Transducer/Ts | PI_R/Integrator
      | (Discrete or Continuous)/Ts | PI_M/Integrator
      | (Discrete or Continuous)/Ts | VRminmax/Ts | K_G//(1+sT_G)/Ts
      mask DialogControl TabGeneral Prompt: physmod:ee:library:comments:control:eeSmST4C:tab_General
      mask DialogControl E_FD0 Prompt: Initial field voltage, Efd0 (pu)
      mask DialogControl V_T0 Prompt: Initial terminal voltage, Vt0 (pu)
      mask DialogControl I_T0 Prompt: Initial terminal current, It0 (pu)
      mask DialogControl Ts Prompt: Sample time (-1 for inherited)
      mask DialogControl TabPrecontrol Prompt: physmod:ee:library:comments:control:eeSmST4C:tab_PreControl
      mask DialogControl T_R Prompt: Regulator input filter time constant, T_R (s)
      mask DialogControl TabControl Prompt: physmod:ee:library:comments:control:eeSmST4C:tab_Control
      mask DialogControl K_PR Prompt: Voltage regulator proportional gain, K_PR (pu)
      mask DialogControl K_IR Prompt: Voltage regulator integral gain, K_IR (pu/s)
      mask DialogControl T_A Prompt: Thyristor bridge firing control equivalent time constant, T_A (s)
      mask DialogControl K_PM Prompt: Forward proportional gain of inner loop field regulator, K_PM (pu)
      mask DialogControl K_IM Prompt: Forward integral gain of inner loop field regulator, K_IM (pu/s)
      mask DialogControl K_G Prompt: Feedback gain of field current regulator, K_G (pu)
      mask DialogControl T_G Prompt: Feedback time constant of field current regulator, T_G (s)
      mask DialogControl TabExciter Prompt: physmod:ee:library:comments:control:eeSmST4C:tab_Exciter
      mask DialogControl K_C Prompt: Rectifier loading factor proportional to commutating reactance, K_C (pu)
      mask DialogControl K_P Prompt: Potential circuit (voltage) gain coefficient, K_P (pu)
      mask DialogControl K_I Prompt: Compound circuit (current) gain coefficient, K_I (pu)
      mask DialogControl X_L Prompt: Reactance associated with potential source, X_L (pu)
      mask DialogControl theta_P Prompt: Potential circuit phase angle (degrees)
      mask Display: %ee.mask.drawSTxC(gcb);
  Gain : Gain  Gain=T_SG.Lmd_pu
  Multiport Switch : MultiPortSwitch  Inputs=4  SaturateOnIntegerOverflow=off  InputSameDT=off
  PSS 2A : Subsystem  Commented=on  mask{ks1=T_SG.PSS.Ks1, ks2=T_SG.PSS.Ks2, ks3=T_SG.PSS.Ks3, T6=T_SG.PSS.T6, T7=T_SG.PSS.T7, Tw1=T_SG.PSS.Tw1, Tw2=T_SG.PSS.Tw2, Tw3=T_SG.PSS.Tw3, Tw4=T_SG.PSS.Tw4, T8=T_SG.PSS.T8, T9=T_SG.PSS.T9, M=T_SG.PSS.M, N=T_SG.PSS.N, T1=T_SG.PSS.T1, T2=T_SG.PSS.T2, T3=T_SG.PSS.T3, T4=T_SG.PSS.T4, hasPSS=hasPSS}
      mask prompts: ks1 "PSS gain, K_S1 (pu)"; ks2 "PSS gain, K_S2 (pu)"; ks3 "PSS gain, K_S3 (pu)"; T6 "PSS transducer time constant, T_6 (s)"; T7 "PSS transducer time constant, T_7 (s)"; Tw1 "PSS washout time constant, T_w1 (s)"; Tw2 "PSS washout time constant, T_w2 (s)"; Tw3 "PSS washout time constant, T_w3 (s)"; Tw4 "PSS washout time constant, T_w4 (s)"; T8 "PSS transducer time constant, T_8 (s)"; T9 "PSS washout time constant, T_9 (s)"; M "Denominator exponent for ramp-track filter, M"; N "Overall exponent for ramp-track filter, N"; T1 "PSS numerator (lead) compensating time constant (first block), T_1 (s)"; T2 "PSS denominator (lag) compensating time constant (first block), T_2 (s)"; T3 "PSS numerator (lead) compensating time constant (second block), T_3 (s)"; T4 "PSS denominator (lag) compensating time constant (second block), T_4 (s)"
      mask init:
      | if hasPSS == 1
      |     pss.Ks1 = 0;
      |     % TO BE CONTINUED
      | end
  Sum : Sum  Inputs=|++
  Sum1 : Sum  Inputs=|++
  Sum2 : Sum  Inputs=|++
  Sum3 : Sum  Inputs=|+-
  Sum6 : Sum  Inputs=|+-
  Switch : Switch  Threshold=1  SaturateOnIntegerOverflow=off  InputSameDT=off
  Terminal voltage magnitude : Subsystem
  Vst : Constant  Value=0
  Out1 : Outport
  wires:
  Constant5/1 -> Sum3/2
  Constant4/1 -> Sum6/2
  Sum3/1 -> PSS 2A/2(Vsi2)  "delta_Te_pu"
  Sum6/1 -> PSS 2A/1(Vsi1)  "delta_w_pu"
  Terminal voltage magnitude/1(Vt) -> Exciter ST1/2(Vt), Exciter ST4B/3(V_T), Exciter AC4A/2(Vt)
  Sum2/1 -> Multiport Switch/4
  Sum1/1 -> Multiport Switch/3
  Sum/1 -> Multiport Switch/2
  Multiport Switch/1 -> Out1/1
  Vd/1 -> Terminal voltage magnitude/2(Vd)
  Ifd_pu/1 -> Gain/1
  Exciter ST1/1(Vfn_pu) -> Sum2/1
  Exciter ST4B/1(Efd_pu) -> Sum1/1
  Constant/1 -> Switch/2
  Vsi2/1 -> Sum3/1
  Exciter AC4A/1(Vfn_pu) -> Sum/1
  Efd0_pu/1 -> Multiport Switch/5, Sum/2, Sum1/2, Sum2/2
  Vq/1 -> Terminal voltage magnitude/1(Vq)
  Vst/1 -> Switch/3  "Vst"
  Switch/1 -> Exciter ST1/3(Vs), Exciter AC4A/3(Vs), Exciter ST4B/2(V_S)
  Vsi1/1 -> Sum6/1
  PSS 2A/1(Vst) -> Switch/1  "Vst"
  V_REF/1 -> Exciter AC4A/1(vref), Exciter ST1/1(vref), Exciter ST4B/1(V_REF)
  Constant1/1 -> Multiport Switch/1
  Gain/1 -> Exciter ST4B/4(Ifd_pu)

== system myLibrary/SG_step/Governor-Turbine ==
  Pref : Inport
  wm : Inport  Port=2
  d_theta : Inport  Port=3
  Constant : Constant  Value=selectGovturb
  IEEEG1 : Subsystem  AncestorBlock=eeGovernorG1/Governor Type 1  LoadFcn=ee_sli_rtmsupport( 'loadfcn', gcbh );  mask(Governor Type 1){pu_speed_reference=1, pu_torque0=initSG.Pm, Ts=-1, K=1/T_SG.mech.R, T_1=initMachineBlocks{SGnum,14}(1), T_2=initMachineBlocks{SGnum,14}(2), T_3=initMachineBlocks{SGnum,14}(3), U_o=inf, U_c=-inf, P_max=1, P_min=0, K_1=initMachineBlocks{SGnum,15}(1), K_3=initMachineBlocks{SGnum,15}(2), K_5=initMachineBlocks{SGnum,15}(3), K_7=initMachineBlocks{SGnum,15}(4), K_2=initMachineBlocks{SGnum,15}(5), K_4=initMachineBlocks{SGnum,15}(6), K_6=initMachineBlocks{SGnum,15}(7), K_8=initMachineBlocks{SGnum,15}(8), T_4=initMachineBlocks{SGnum,15}(9), T_5=initMachineBlocks{SGnum,15}(10), T_6=initMachineBlocks{SGnum,15}(11), T_7=initMachineBlocks{SGnum,15}(12), db1=1}
      mask prompts: pu_speed_reference "physmod:ee:library:comments:control:eeGovernorG1:SpeedReferencepu_MP"; pu_torque0 "physmod:ee:library:comments:control:eeGovernorG1:InitialTorquepu_MP"; Ts "physmod:ee:library:comments:control:eeGovernorG1:SampleTime1ForInherited_MP"; K "physmod:ee:library:comments:control:eeGovernorG1:GovernorGain1droopKpu_MP"; T_1 "physmod:ee:library:comments:control:eeGovernorG1:LagTimeConstantT_1s_MP"; T_2 "physmod:ee:library:comments:control:eeGovernorG1:LeadTimeConstantT_2s_MP"; T_3 "physmod:ee:library:comments:control:eeGovernorG1:ValvePositionTimeConstantT_3s_MP"; U_o "physmod:ee:library:comments:control:eeGovernorG1:MaximumValveOpeningRateU_opus_MP"; U_c "physmod:ee:library:comments:control:eeGovernorG1:MaximumValveClosingRateU_cpus_MP"; P_max "physmod:ee:library:comments:control:eeGovernorG1:MaximumValveOpeningOnMWCapabilityP_maxpu_MP"; P_min "physmod:ee:library:comments:control:eeGovernorG1:MinimumValveOpeningOnMWCapabilityP_minpu_MP"; K_1 "physmod:ee:library:comments:control:eeGovernorG1:HPFractionK_1_MP"; K_3 "physmod:ee:library:comments:control:eeGovernorG1:HPFractionK_3_MP"; K_5 "physmod:ee:library:comments:control:eeGovernorG1:HPFractionK_5_MP"; K_7 "physmod:ee:library:comments:control:eeGovernorG1:HPFractionK_7_MP"; K_2 "physmod:ee:library:comments:control:eeGovernorG1:LPFractionK2_MP"; K_4 "physmod:ee:library:comments:control:eeGovernorG1:LPFractionK_4_MP"; K_6 "physmod:ee:library:comments:control:eeGovernorG1:LPFractionK_6_MP"; K_8 "physmod:ee:library:comments:control:eeGovernorG1:LPFractionK_8_MP"; T_4 "physmod:ee:library:comments:control:eeGovernorG1:TimeConstantForSteamInletT_4s_MP"; T_5 "physmod:ee:library:comments:control:eeGovernorG1:TimeConstantForSecondBoilerPassT_5s_MP"; T_6 "physmod:ee:library:comments:control:eeGovernorG1:TimeConstantForThirdBoilerPassT_6s_MP"; T_7 "physmod:ee:library:comments:control:eeGovernorG1:TimeConstantForFourthBoilerPassT_7s_MP"; db1 "physmod:ee:library:comments:control:eeGovernorG1:Deadband_MP"
      mask help: physmod:ee:library:comments:control:eeGovernorG1:GovernorType1_MD
      mask init:
      | timeDomain = ee.mask.getTimeDomain(Ts);
      settings: LibrarySourceBlock=eeGovernorG1/Governor Type 1  CopyFcn=ee_sli_rtmsupport( 'copyfcn', gcbh );  DeleteFcn=ee_sli_rtmsupport( 'deletefcn', gcbh );  ModelCloseFcn=ee_sli_rtmsupport( 'modelclosefcn', gcbh );  PostSaveFcn=ee_sli_rtmsupport( 'postsavefcn', gcbh );  PreCopyFcn=ee_sli_rtmsupport( 'precopyfcn', gcbh );  OpenFcn=ee_sli_rtmsupport( 'openfcn', gcbh );  CloseFcn=ee_sli_rtmsupport( 'closefcn', gcbh );  PreDeleteFcn=ee_sli_rtmsupport( 'predeletefcn', gcbh );
      mask Help: web(nesl_help(gcbh))
      mask TypeOptions Ts:
      | Lead-Lag/Ts | Low-Pass Filter/Ts | Low-Pass Filter1/Ts | Low-Pass Filter2/Ts | Low-Pass Filter3/Ts | Integrator
      | (Discrete or Continuous)/Ts
      mask DialogControl TabGeneral Prompt: physmod:ee:library:comments:control:eeGovernorG1:tab_General
      mask DialogControl pu_speed_reference Prompt: Speed reference (pu)
      mask DialogControl pu_torque0 Prompt: Initial torque (pu)
      mask DialogControl Ts Prompt: Sample time (-1 for inherited)
      mask DialogControl TabGovernor Prompt: physmod:ee:library:comments:control:eeGovernorG1:tab_Governor
      mask DialogControl K Prompt: Governor gain (1/droop), K (pu)
      mask DialogControl T_1 Prompt: Lag time constant, T_1 (s)
      mask DialogControl T_2 Prompt: Lead time constant, T_2 (s)
      mask DialogControl T_3 Prompt: Valve position time constant, T_3 (s)
      mask DialogControl U_o Prompt: Maximum valve opening rate, U_o (pu/s)
      mask DialogControl U_c Prompt: Maximum valve closing rate, U_c (pu/s)
      mask DialogControl P_max Prompt: Maximum valve opening, on MW capability, P_max (pu)
      mask DialogControl P_min Prompt: Minimum valve opening, on MW capability, P_min (pu)
      mask DialogControl K_1 Prompt: HP fraction, K_1
      mask DialogControl K_3 Prompt: HP fraction, K_3
      mask DialogControl K_5 Prompt: HP fraction, K_5
      mask DialogControl K_7 Prompt: HP fraction, K_7
      mask DialogControl K_2 Prompt: LP fraction, K2
      mask DialogControl K_4 Prompt: LP fraction, K_4
      mask DialogControl K_6 Prompt: LP fraction, K_6
      mask DialogControl K_8 Prompt: LP fraction, K_8
      mask DialogControl T_4 Prompt: Time constant for steam inlet, T_4 (s)
      mask DialogControl T_5 Prompt: Time constant for second boiler pass, T_5 (s)
      mask DialogControl T_6 Prompt: Time constant for third boiler pass, T_6 (s)
      mask DialogControl T_7 Prompt: Time constant for fourth boiler pass, T_7 (s)
      mask DialogControl db1 Prompt: Deadband
  Multiport Switch1 : MultiPortSwitch  SaturateOnIntegerOverflow=off  InputSameDT=off
  Steam Turbine and Governor : Subsystem  Commented=on  DialogController=POWERSYS.PowerSysDialog  mask(Steam Turbine and Governor){gentype=Tandem-compound (multi-mass), reg1=[ 1  T_SG.mech.R   0 ], reg2=[ 0  1], reg3=[ -inf  inf  0  inf], N=T_SG.fb*60, turb1=initMachineBlocks{SGnum,8}, turb2=initMachineBlocks{SGnum,9}, HA=initMachineBlocks{SGnum,10}, KA=initMachineBlocks{SGnum,11}, DA=initMachineBlocks{SGnum,12}, ini1=1.003, ini2=initMachineBlocks{SGnum,7}}
      mask prompts: gentype "Generator type"; reg1 "Regulator gain, perm. droop, dead zone [ Kp  Rp(pu)  Dz(pu) ]:"; reg2 "Speed relay and servo-motor time constants [ Tsr  Tsm ] (s):"; reg3 "Gate opening limits [ vgmin,vgmax (pu/s)  gmin,gmax (pu)]:"; N "Nominal speed of synchronous machine (rpm)"; turb1 "Steam turbine time constants [ T2  T3  T4  T5 ] (s):"; turb2 "Turbine torque fractions [ F2  F3  F4  F5 ]:"; HA "Coeff. of inertia [ H2  H3  H4  H5 ] (s):"; KA "Stiffness coeff. [ K12  K23  K34  K45 ] (pu/rad):"; DA "Damping factors [ D2  D3  D4  D5 ] (pu T/pu dw):"; ini1 "Initial power Pm0 (pu):"; ini2 "Initial power and generator rotor angle [ Pm0 (pu)  th0(deg) ]:"
      mask help:
      | Implements a complete tandem-compound steam prime mover system, including
      | speed regulator, steam turbine and a shaft with up to 4 masses. The genererator's
      | mass is labelled mass #1 and is not included here. The shaft mass closest to the
      | generator is #2, the farthest is #5. If a mass is not to be included, set it's inertia H to
      | zero. The damping factor and rigidity coefficients corresponding to omitted masses
      | are not considered and can be left as is. When masses are omitted, the remaining
      | system is "compressed" towards the generator i.e. if only 2 masses are used, it will
      | be masses #2 and #3. The input data for the masses considered is shifted accordingly.
      mask init: same as myLibrary/SG/Governor-Turbine/Steam Turbine and Governor
      settings: OpenFcn=sps_rtmsupport('OpenFcn',gcbh)
      mask Help: helpview(psbhelp);
      mask TypeOptions gentype: Tandem-compound (single mass) | Tandem-compound (multi-mass)
      mask Callback gentype: powericon('psbcallbacks',gcbh,'SteamTurbine');
      mask Display: %plot([0 0],[t t])
  Terminator1 : Terminator
  Terminator2 : Terminator
  Terminator3 : Terminator  Commented=on
  Terminator4 : Terminator  Commented=on
  Terminator5 : Terminator  Commented=on
  w_ref : Constant
  Pm : Outport
  wires:
  Steam Turbine and Governor/4(Pm) -> Multiport Switch1/3  "Pm"
  Steam Turbine and Governor/1(dw_5-2) -> Terminator5/1
  Steam Turbine and Governor/3(gate) -> Terminator3/1
  Steam Turbine and Governor/2(Tr5-2) -> Terminator4/1
  w_ref/1 -> Steam Turbine and Governor/1(wref)
  d_theta/1 -> Steam Turbine and Governor/4(d_theta)
  wm/1 -> Steam Turbine and Governor/3(wm), IEEEG1/1(speed_pu)
  IEEEG1/3(Pm) -> Multiport Switch1/2
  Constant/1 -> Multiport Switch1/1
  Multiport Switch1/1 -> Pm/1
  IEEEG1/2(Pm(LP)) -> Terminator2/1
  IEEEG1/1(Pm(HP)) -> Terminator1/1
  Pref/1 -> IEEEG1/2(Pref), Steam Turbine and Governor/2(Pref), Multiport Switch1/4

== system myLibrary/SG_step/Vector magnitude  ==
  Vq : Inport
  Vd : Inport  Port=2
  Add10 : Sum
  Product : Product
  Product1 : Product
  Square Root : Sqrt
  V : Outport
  wires:
  Square Root/1 -> V/1  "V"
  Vq/1 -> Product/2, Product/1
  Add10/1 -> Square Root/1
  Product1/1 -> Add10/2
  Vd/1 -> Product1/1, Product1/2
  Product/1 -> Add10/1

== system myLibrary/qd transform/qd0 Transformation ==
  a : Inport
  b : Inport  Port=2
  c : Inport  Port=3
  Angle : Inport  Port=4
  Demux1 : Demux  Outputs=3
  Matriu T : Subsystem
  Mux : Mux  Inputs=3
  Product : Product  Multiplication=Matrix(*)
  Terminator : Terminator
  q : Outport  VectorParamsAs1DForOutWhenUnconnected=off
  d : Outport  Port=2  VectorParamsAs1DForOutWhenUnconnected=off
  wires:
  Product/1 -> Demux1/1
  Matriu T/1(Out1) -> Product/1
  Demux1/1 -> q/1
  Demux1/2 -> d/1
  Demux1/3 -> Terminator/1
  Angle/1 -> Matriu T/1(u)
  Mux/1 -> Product/2
  a/1 -> Mux/1
  b/1 -> Mux/2
  c/1 -> Mux/3

== system myLibrary/GFOL/Control/Active Power Control ==
  Pac_ref : Inport
  w : Inport  Port=2
  id : Inport  Port=3
  iq : Inport  Port=4
  Ud : Inport  Port=5
  Uq : Inport  Port=6
  Constant : Constant  Value=T_VSC.wb
  Gain : Gain  Gain=3/2
  Integrator : Integrator  InitialCondition=initVSC.idiffq
  Ki : Gain  Gain=T_VSC.ki_P
  Kp : Gain  Gain=T_VSC.kp_P
  Low-Pass Filter (Discrete or Continuous)4 : eeGeneralControl/Low-Pass Filter (Discrete or Continuous)  K=1  T=T_VSC.tau_droop_f  B=inf  A=-inf  init_option=Specify as parameter  x0=T_VSC.wb  Ts=-1
  Product1 : Product
  Product3 : Product
  Scope : Scope  NumInputPorts=2
  Sum : Sum  Inputs=+-+
  Sum1 : Sum
  Sum2 : Sum  Inputs=|+-
  Sum4 : Sum
  droop : Gain  Gain=T_VSC.k_droop_f/T_VSC.wb
  Iq_ref : Outport
  wires:
  droop/1 -> Sum/3
  w/1 -> Low-Pass Filter (Discrete or Continuous)4/1
  Constant/1 -> Sum2/1
  Sum2/1 -> droop/1
  Low-Pass Filter (Discrete or Continuous)4/1 -> Sum2/2
  Uq/1 -> Product3/1
  iq/1 -> Product3/2
  Ud/1 -> Product1/1
  id/1 -> Product1/2
  Product3/1 -> Sum1/1
  Product1/1 -> Sum1/2
  Sum1/1 -> Gain/1
  Pac_ref/1 -> Scope/1, Sum/1
  Gain/1 -> Scope/2, Sum/2
  Integrator/1 -> Sum4/1
  Kp/1 -> Sum4/2
  Ki/1 -> Integrator/1
  Sum/1 -> Ki/1, Kp/1
  Sum4/1 -> Iq_ref/1

== system myLibrary/GFOL/Control/Clarke Anti-Transformation ==
  V_alfa_diff : Inport
  V_beta_dfff : Inport  Port=2
  V_0_diff : Inport  Port=3
  Constant{,2,5,8} (4 alike) : Constant
  Constant1 : Constant  Value=0
  Constant3 : Constant  Value=-1/2
  Constant4 : Constant  Value=-sqrt(3)/2
  Constant6 : Constant  Value=-1/2
  Constant7 : Constant  Value=sqrt(3)/2
  Demux : Demux  Outputs=3
  Display : Display
  Math Function : Math  Operator=transpose  SignedPower=on
  Matrix Concatenate : Concatenate  NumInputs=3  Mode=Multidimensional array  ConcatenateDimension=2
  Mux{,1..3} (4 alike) : Mux  Inputs=3
  Product : Product  Multiplication=Matrix(*)
  Va_diff : Outport  VectorParamsAs1DForOutWhenUnconnected=off
  Vb_diff : Outport  Port=2  VectorParamsAs1DForOutWhenUnconnected=off
  Vc_diff : Outport  Port=3  VectorParamsAs1DForOutWhenUnconnected=off
  wires:
  Constant/1 -> Mux1/1
  Constant1/1 -> Mux1/2
  Constant2/1 -> Mux1/3
  Constant3/1 -> Mux2/1
  Constant4/1 -> Mux2/2
  Constant5/1 -> Mux2/3
  Constant6/1 -> Mux3/1
  Constant7/1 -> Mux3/2
  Constant8/1 -> Mux3/3
  Matrix Concatenate/1 -> Math Function/1
  Mux2/1 -> Matrix Concatenate/2
  Mux3/1 -> Matrix Concatenate/3
  Mux1/1 -> Matrix Concatenate/1
  Product/1 -> Demux/1
  Demux/1 -> Va_diff/1  "Va"
  Demux/2 -> Vb_diff/1  "Vb"
  Demux/3 -> Vc_diff/1  "Vc"
  Mux/1 -> Product/2
  Math Function/1 -> Display/1, Product/1
  V_alfa_diff/1 -> Mux/1  "Valfa"
  V_beta_dfff/1 -> Mux/2  "Vbeta"
  V_0_diff/1 -> Mux/3  "0"
